simulink model "VHF_central_unit"  (R2024a)
settings: Solver=FixedStepDiscrete  StartTime=0.0  StopTime=10.0  FixedStep=0.001  RelTol=1e-3  EnableMultiTasking=on
PreLoadFcn:
  | try
  | MDL_install;
  | catch
  | end
InitFcn:
  | EcoCoder_PreCheckLic();
undefined symbols (not defined in the file or in its folder): C_ROTSPD_ZERO, C_SOC_ZERO, h, km, s, V
libraries: CoderSF_BSW_Libs x222, SF_CanService_Libs x16, CoderSF_ADC2Volt_Libs x6, CoderSF_6AxisMEMS_Libs x6, canmsglib x3, EV_ASWLibs x2, simulink x2, Chassis_stability_controllers x1, CoderSF_KeyCycle_Libs x1
(part 2 of 4)

== system VHF_central_unit/General Power Control1/Control KeyCycle ==
  flgKeyon_raw : Inport
  function : TriggerPort  TriggerType=function-call  VariantControl=(inherit)
  KeyCycle to Reset : CoderSF_KeyCycle_Libs/KeyCycle to Reset
  Read Calibration1 : CoderSF_BSW_Libs/Calibration & Measurement/Read Calibration  variable_name=PwrMCU_tResetDbncKeyOffFall_val  variable_value=0.2  variable_type=single  variable_min=[]  variable_max=[]  unitStr=s  descStr=""
      settings: AttributesFormatString=value:%<variable_value> type:%<variable_type> max:%<variable_max> Min:%<variable_min>
  Read Calibration2 : CoderSF_BSW_Libs/Calibration & Measurement/Read Calibration  variable_name=PwrMCU_tResetDbncKeyOffRise_val  variable_value=0.2  variable_type=single  variable_min=[]  variable_max=[]  unitStr=s  descStr=""
      settings: AttributesFormatString=value:%<variable_value> type:%<variable_type> max:%<variable_max> Min:%<variable_min>
  Read Calibration3 : CoderSF_BSW_Libs/Calibration & Measurement/Read Calibration  variable_name=PwrMCU_flgResetSWEn_val  variable_value=0  variable_type=boolean  variable_min=[]  variable_max=[]  unitStr=""  descStr=""
      settings: AttributesFormatString=value:%<variable_value> type:%<variable_type> max:%<variable_max> Min:%<variable_min>
  flgReset : Outport
  wires:
  flgKeyon_raw/1 -> KeyCycle to Reset/1
  Read Calibration2/1 -> KeyCycle to Reset/4
  Read Calibration3/1 -> KeyCycle to Reset/2
  Read Calibration1/1 -> KeyCycle to Reset/3
  KeyCycle to Reset/1 -> flgReset/1

== system VHF_central_unit/General Power Control1/Control Restore All NVM Data ==
  flgEnNVMRestore : Inport
  function : TriggerPort  TriggerType=function-call  VariantControl=(inherit)
  Restore All NVM Data Hold : CoderSF_BSW_Libs/Non-volatile Memory Blocks/Restore All NVM Data Hold
  wires:
  flgEnNVMRestore/1 -> Restore All NVM Data Hold/Enable

== system VHF_central_unit/General Power Control1/Debounce KeyOn ==
  flgKeyOnRaw : Inport
  function : TriggerPort  TriggerType=function-call  VariantControl=(inherit)
  Falling Edge Debounce1 : CoderSF_BSW_Libs/Application Base Blocks/Falling Edge Debounce  ic=off
  Read Calibration3 : CoderSF_BSW_Libs/Calibration & Measurement/Read Calibration  variable_name=PwrMCU_tDbncKeyOn_val  variable_value=0.05  variable_type=single  variable_min=[]  variable_max=[]  unitStr=s  descStr=""
      settings: AttributesFormatString=value:%<variable_value> type:%<variable_type> max:%<variable_max> Min:%<variable_min>
  Read Calibration5 : CoderSF_BSW_Libs/Calibration & Measurement/Read Calibration  variable_name=PwrMCU_tDbncKeyOff_val  variable_value=0.05  variable_type=single  variable_min=[]  variable_max=[]  unitStr=s  descStr=""
      settings: AttributesFormatString=value:%<variable_value> type:%<variable_type> max:%<variable_max> Min:%<variable_min>
  Rising Edge Debounce : CoderSF_BSW_Libs/Application Base Blocks/Rising Edge Debounce  ic=off
  Write and Read Measurement : CoderSF_BSW_Libs/Calibration & Measurement/Write and Read Measurement  variable_name=PwrMCU_flgKeyOnDbnc  variable_value=0  variable_type=boolean  numD=1  unitStr=""  descStr=""
      settings: AttributesFormatString=type:%<variable_type> Dimensions:%<numD>
  PwrMCU_flgKeyOnDbnc : Outport
  wires:
  Read Calibration5/1 -> Falling Edge Debounce1/1
  Read Calibration3/1 -> Rising Edge Debounce/1
  Rising Edge Debounce/1 -> Falling Edge Debounce1/2
  Falling Edge Debounce1/1 -> Write and Read Measurement/1
  Write and Read Measurement/1 -> PwrMCU_flgKeyOnDbnc/1  "PwrMCU_flgKeyOnDbnc"
  flgKeyOnRaw/1 -> Rising Edge Debounce/2

== system VHF_central_unit/General Power Control1/Enable Restore And Store NVM ==
  flgKeyon : Inport
  flgEnRestoreStoreNVM_val : Inport  Port=2
  function : TriggerPort  TriggerType=function-call  VariantControl=(inherit)
  Constant2 : Constant  Value=0
  Logical Operator2 : Logic  AllPortsSameDT=off  OutDataTypeStr=boolean
  SR Flip Flop : CoderSF_BSW_Libs/Application Base Blocks/SR Flip Flop
  Terminator : Terminator
  flgEnStoreNVM : Outport
  wires:
  flgKeyon/1 -> SR Flip Flop/1
  Logical Operator2/1 -> flgEnStoreNVM/1
  Constant2/1 -> SR Flip Flop/2
  SR Flip Flop/1 -> Logical Operator2/1
  flgEnRestoreStoreNVM_val/1 -> Logical Operator2/2
  SR Flip Flop/2 -> Terminator/1

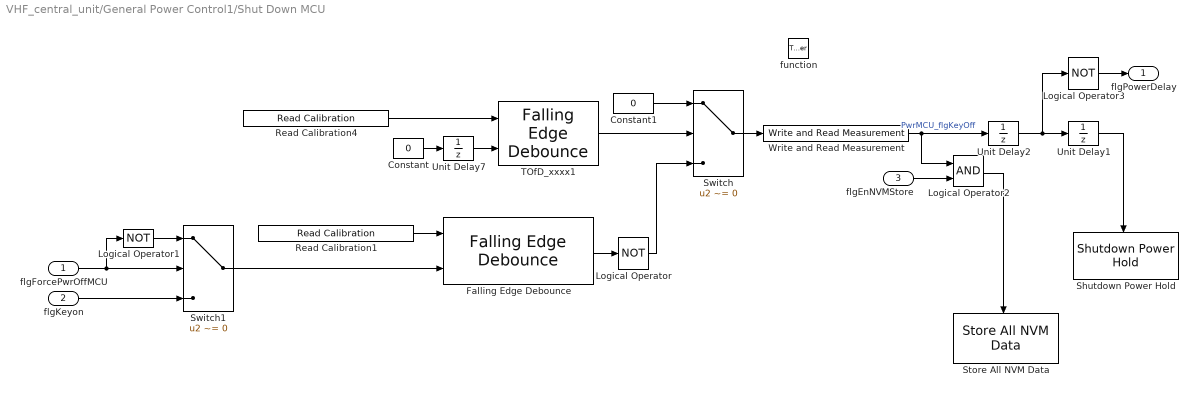
== system VHF_central_unit/General Power Control1/Shut Down MCU ==
  flgForcePwrOffMCU : Inport
  flgKeyon : Inport  Port=2
  flgEnNVMStore : Inport  Port=3
  function : TriggerPort  TriggerType=function-call  VariantControl=(inherit)
  Constant : Constant  Value=0
  Constant1 : Constant  Value=0  OutDataTypeStr=Inherit: Inherit via back propagation  SampleTime=-1
  Falling Edge Debounce : CoderSF_BSW_Libs/Application Base Blocks/Falling Edge Debounce  ic=off
  Logical Operator : Logic  Operator=NOT  AllPortsSameDT=off  OutDataTypeStr=boolean
  Logical Operator1 : Logic  Operator=NOT  AllPortsSameDT=off  OutDataTypeStr=boolean
  Logical Operator2 : Logic  AllPortsSameDT=off  OutDataTypeStr=boolean
  Logical Operator3 : Logic  Operator=NOT  AllPortsSameDT=off  OutDataTypeStr=boolean
  Read Calibration1 : CoderSF_BSW_Libs/Calibration & Measurement/Read Calibration  variable_name=PwrMCU_tShutDownDelay_val  variable_value=0.5  variable_type=single  variable_min=[]  variable_max=[]  unitStr=s  descStr=""
      settings: AttributesFormatString=value:%<variable_value> type:%<variable_type> max:%<variable_max> Min:%<variable_min>
  Read Calibration4 : CoderSF_BSW_Libs/Calibration & Measurement/Read Calibration  variable_name=PwrMCU_tWaitKeyOn_val  variable_value=0.2  variable_type=single  variable_min=[]  variable_max=[]  unitStr=s  descStr=""
      settings: AttributesFormatString=value:%<variable_value> type:%<variable_type> max:%<variable_max> Min:%<variable_min>
  Shutdown Power Hold : CoderSF_BSW_Libs/System Management Blocks/Shutdown Power Hold  tWait_ms=500
  Store All NVM Data : CoderSF_BSW_Libs/Non-volatile Memory Blocks/Store All NVM Data  TriggerTypeSet=rising
  Switch : Switch  Criteria=u2 ~= 0  SaturateOnIntegerOverflow=off  InputSameDT=off
  Switch1 : Switch  Criteria=u2 ~= 0  SaturateOnIntegerOverflow=off  InputSameDT=off
  TOfD_xxxx1 : CoderSF_BSW_Libs/Application Base Blocks/Falling Edge Debounce  ic=off
  Unit Delay1 : UnitDelay  SampleTime=-1
      settings: AttributesFormatString=InitialCondition:%<InitialCondition>
  Unit Delay2 : UnitDelay  SampleTime=-1
      settings: AttributesFormatString=InitialCondition:%<InitialCondition>
  Unit Delay7 : UnitDelay  InitialCondition=1  SampleTime=-1
      settings: AttributesFormatString=InitialCondition:%<InitialCondition>
  Write and Read Measurement : CoderSF_BSW_Libs/Calibration & Measurement/Write and Read Measurement  variable_name=PwrMCU_flgKeyOff  variable_value=0  variable_type=boolean  numD=1  unitStr=""  descStr=""
      settings: AttributesFormatString=type:%<variable_type> Dimensions:%<numD>
  flgPowerDelay : Outport
  wires:
  Logical Operator3/1 -> flgPowerDelay/1
  Unit Delay2/1 -> Unit Delay1/1, Logical Operator3/1
  Read Calibration1/1 -> Falling Edge Debounce/1
  Logical Operator/1 -> Switch/3
  Falling Edge Debounce/1 -> Logical Operator/1
  Constant1/1 -> Switch/1
  TOfD_xxxx1/1 -> Switch/2
  flgKeyon/1 -> Switch1/3
  Read Calibration4/1 -> TOfD_xxxx1/1
  Unit Delay7/1 -> TOfD_xxxx1/2
  Constant/1 -> Unit Delay7/1
  flgForcePwrOffMCU/1 -> Switch1/2, Logical Operator1/1
  Switch1/1 -> Falling Edge Debounce/2
  Logical Operator1/1 -> Switch1/1
  Unit Delay1/1 -> Shutdown Power Hold/Enable
  Switch/1 -> Write and Read Measurement/1
  Logical Operator2/1 -> Store All NVM Data/Trigger
  flgEnNVMStore/1 -> Logical Operator2/2
  Write and Read Measurement/1 -> Unit Delay2/1, Logical Operator2/1  "PwrMCU_flgKeyOff"

== system VHF_central_unit/Get wake-up signal1/Get wake-up signal ==
  function : TriggerPort  TriggerType=function-call  VariantControl=(inherit)
  ADC Value To Volt : CoderSF_ADC2Volt_Libs/ADC Value To Volt  ResValue=12  RefValue=5  TypeOut=Inherit: Inherit via back propagation  WithDiv=on  DivValue=3.48  SerValue=22
  Hysteresis : CoderSF_BSW_Libs/Application Base Blocks/Hysteresis
  Logical Operator : Logic  Operator=OR  Inputs=3  AllPortsSameDT=off  OutDataTypeStr=boolean
  Read ADC Value : CoderSF_BSW_Libs/ADC/Read ADC Value  channel=AI_KEYON
  Read Calibration1 : CoderSF_BSW_Libs/Calibration & Measurement/Read Calibration  variable_name=PwrMCU_voltKeyOnHysteresis_val  variable_value=3  variable_type=single  variable_min=[]  variable_max=[]  unitStr=s  descStr=""
      settings: AttributesFormatString=value:%<variable_value> type:%<variable_type> max:%<variable_max> Min:%<variable_min>
  Read Calibration5 : CoderSF_BSW_Libs/Calibration & Measurement/Read Calibration  variable_name=PwrMCU_voltKeyOffThreshold_val  variable_value=2  variable_type=single  variable_min=[]  variable_max=[]  unitStr=s  descStr=""
      settings: AttributesFormatString=value:%<variable_value> type:%<variable_type> max:%<variable_max> Min:%<variable_min>
  Switch Input1 : CoderSF_BSW_Libs/Digital I//O/Switch Input  portNum=DI_WAKE1
  Switch Input2 : CoderSF_BSW_Libs/Digital I//O/Switch Input  portNum=DI_WAKE2
  Write and Read Measurement : CoderSF_BSW_Libs/Calibration & Measurement/Write and Read Measurement  variable_name=PwrMCU_voltKeyOn  variable_value=0  variable_type=single  numD=1  unitStr=V  descStr=""
      settings: AttributesFormatString=type:%<variable_type> Dimensions:%<numD>
  Write and Read Measurement1 : CoderSF_BSW_Libs/Calibration & Measurement/Write and Read Measurement  variable_name=PwrMCU_adKeyOn  variable_value=0  variable_type=uint16  numD=1  unitStr=""  descStr=""
      settings: AttributesFormatString=type:%<variable_type> Dimensions:%<numD>
  Write and Read Measurement2 : CoderSF_BSW_Libs/Calibration & Measurement/Write and Read Measurement  variable_name=PwrMCU_flgKeyOnRead  variable_value=0  variable_type=boolean  numD=1  unitStr=""  descStr=""
      settings: AttributesFormatString=type:%<variable_type> Dimensions:%<numD>
  PwrVCU_flgKeyOn : Outport
  wires:
  Logical Operator/1 -> PwrVCU_flgKeyOn/1
  Hysteresis/1 -> Write and Read Measurement2/1
  Switch Input1/1 -> Logical Operator/2
  Switch Input2/1 -> Logical Operator/3
  Read ADC Value/1 -> Write and Read Measurement1/1
  ADC Value To Volt/1 -> Write and Read Measurement/1
  Read Calibration5/1 -> Hysteresis/3
  Read Calibration1/1 -> Hysteresis/1
  Write and Read Measurement/1 -> Hysteresis/2  "PwrMCU_voltKeyOn"
  Write and Read Measurement1/1 -> ADC Value To Volt/1  "PwrMCU_adKeyOn"
  Write and Read Measurement2/1 -> Logical Operator/1  "PwrMCU_flgKeyOnRead"

== system VHF_central_unit/MEMS sensor/Sensor Self Test ==
  function : TriggerPort  TriggerType=function-call  VariantControl=(inherit)
  6-Axis MEMS Sensor Self Test : CoderSF_6AxisMEMS_Libs/6-Axis MEMS Sensor/6-Axis MEMS Sensor Self Test
  "Write Fixed NVM " : CoderSF_BSW_Libs/Non-volatile Memory Blocks/Write Fixed NVM   data_name=Fnvm_Sensor_stSelfTest
  Write and Read Measurement : CoderSF_BSW_Libs/Calibration & Measurement/Write and Read Measurement  variable_name=Sensor_stSelfTest  variable_value=0  variable_type=uint8  numD=1  unitStr=""  descStr=""
      settings: AttributesFormatString=type:%<variable_type> Dimensions:%<numD>
  wires:
  6-Axis MEMS Sensor Self Test/1 -> Write and Read Measurement/1
  Write and Read Measurement/1 -> "Write Fixed NVM "/1  "Sensor_stSelfTest"

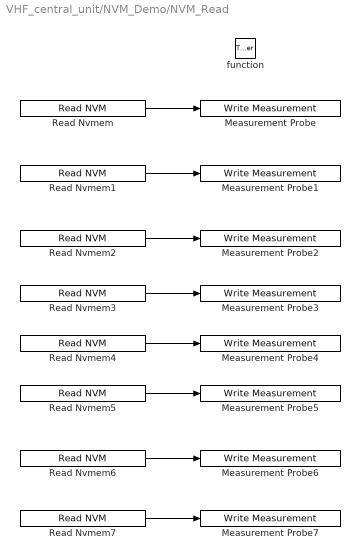
== system VHF_central_unit/NVM_Demo/NVM_Read ==
  function : TriggerPort  TriggerType=function-call  VariantControl=(inherit)
  Measurement Probe : CoderSF_BSW_Libs/Calibration & Measurement/Write Measurement  variable_name=ASW_V_single  variable_value=0  variable_type=single  numD=1  unitStr=""  descStr=""
      settings: AttributesFormatString=value:%<variable_value> type:%<variable_type>
  Measurement Probe1 : CoderSF_BSW_Libs/Calibration & Measurement/Write Measurement  variable_name=ASW_V_int8  variable_value=0  variable_type=int8  numD=1  unitStr=""  descStr=""
      settings: AttributesFormatString=value:%<variable_value> type:%<variable_type>
  Measurement Probe2 : CoderSF_BSW_Libs/Calibration & Measurement/Write Measurement  variable_name=ASW_V_uint8  variable_value=0  variable_type=uint8  numD=1  unitStr=""  descStr=""
      settings: AttributesFormatString=value:%<variable_value> type:%<variable_type>
  Measurement Probe3 : CoderSF_BSW_Libs/Calibration & Measurement/Write Measurement  variable_name=ASW_V_int16  variable_value=0  variable_type=int16  numD=1  unitStr=""  descStr=""
      settings: AttributesFormatString=value:%<variable_value> type:%<variable_type>
  Measurement Probe4 : CoderSF_BSW_Libs/Calibration & Measurement/Write Measurement  variable_name=ASW_V_uint16  variable_value=0  variable_type=uint16  numD=1  unitStr=""  descStr=""
      settings: AttributesFormatString=value:%<variable_value> type:%<variable_type>
  Measurement Probe5 : CoderSF_BSW_Libs/Calibration & Measurement/Write Measurement  variable_name=ASW_V_int32  variable_value=0  variable_type=int32  numD=1  unitStr=""  descStr=""
      settings: AttributesFormatString=value:%<variable_value> type:%<variable_type>
  Measurement Probe6 : CoderSF_BSW_Libs/Calibration & Measurement/Write Measurement  variable_name=ASW_V_uint32  variable_value=0  variable_type=uint32  numD=1  unitStr=""  descStr=""
      settings: AttributesFormatString=value:%<variable_value> type:%<variable_type>
  Measurement Probe7 : CoderSF_BSW_Libs/Calibration & Measurement/Write Measurement  variable_name=ASW_V_boolean  variable_value=0  variable_type=boolean  numD=1  unitStr=""  descStr=""
      settings: AttributesFormatString=value:%<variable_value> type:%<variable_type>
  Read Nvmem : CoderSF_BSW_Libs/Non-volatile Memory Blocks/Read NVM  variable_name=ASW_Nvm_single  variable_type=Inherit from 'Variable definition'
      settings: AttributesFormatString=type:%<variable_type>
  Read Nvmem1 : CoderSF_BSW_Libs/Non-volatile Memory Blocks/Read NVM  variable_name=ASW_Nvm_int8  variable_type=Inherit from 'Variable definition'
      settings: AttributesFormatString=type:%<variable_type>
  Read Nvmem2 : CoderSF_BSW_Libs/Non-volatile Memory Blocks/Read NVM  variable_name=ASW_Nvm_uint8  variable_type=Inherit from 'Variable definition'
      settings: AttributesFormatString=type:%<variable_type>
  Read Nvmem3 : CoderSF_BSW_Libs/Non-volatile Memory Blocks/Read NVM  variable_name=ASW_Nvm_int16  variable_type=Inherit from 'Variable definition'
      settings: AttributesFormatString=type:%<variable_type>
  Read Nvmem4 : CoderSF_BSW_Libs/Non-volatile Memory Blocks/Read NVM  variable_name=ASW_Nvm_uint16  variable_type=Inherit from 'Variable definition'
      settings: AttributesFormatString=type:%<variable_type>
  Read Nvmem5 : CoderSF_BSW_Libs/Non-volatile Memory Blocks/Read NVM  variable_name=ASW_Nvm_int32  variable_type=Inherit from 'Variable definition'
      settings: AttributesFormatString=type:%<variable_type>
  Read Nvmem6 : CoderSF_BSW_Libs/Non-volatile Memory Blocks/Read NVM  variable_name=ASW_Nvm_uint32  variable_type=Inherit from 'Variable definition'
      settings: AttributesFormatString=type:%<variable_type>
  Read Nvmem7 : CoderSF_BSW_Libs/Non-volatile Memory Blocks/Read NVM  variable_name=ASW_Nvm_boolean  variable_type=Inherit from 'Variable definition'
      settings: AttributesFormatString=type:%<variable_type>
  wires:
  Read Nvmem7/1 -> Measurement Probe7/1
  Read Nvmem6/1 -> Measurement Probe6/1
  Read Nvmem5/1 -> Measurement Probe5/1
  Read Nvmem4/1 -> Measurement Probe4/1
  Read Nvmem3/1 -> Measurement Probe3/1
  Read Nvmem2/1 -> Measurement Probe2/1
  Read Nvmem1/1 -> Measurement Probe1/1
  Read Nvmem/1 -> Measurement Probe/1

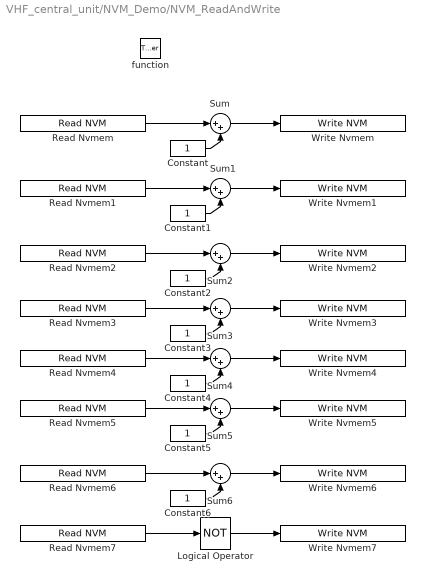
== system VHF_central_unit/NVM_Demo/NVM_ReadAndWrite ==
  function : TriggerPort  TriggerType=function-call  VariantControl=(inherit)
  Constant{,1..6} (7 alike) : Constant  OutDataTypeStr=Inherit: Inherit via back propagation  SampleTime=-1
  Logical Operator : Logic  Operator=NOT  AllPortsSameDT=off  OutDataTypeStr=boolean
  Read Nvmem : CoderSF_BSW_Libs/Non-volatile Memory Blocks/Read NVM  variable_name=ASW_Nvm_single  variable_type=Inherit from 'Variable definition'
      settings: AttributesFormatString=type:%<variable_type>
  Read Nvmem1 : CoderSF_BSW_Libs/Non-volatile Memory Blocks/Read NVM  variable_name=ASW_Nvm_int8  variable_type=Inherit from 'Variable definition'
      settings: AttributesFormatString=type:%<variable_type>
  Read Nvmem2 : CoderSF_BSW_Libs/Non-volatile Memory Blocks/Read NVM  variable_name=ASW_Nvm_uint8  variable_type=Inherit from 'Variable definition'
      settings: AttributesFormatString=type:%<variable_type>
  Read Nvmem3 : CoderSF_BSW_Libs/Non-volatile Memory Blocks/Read NVM  variable_name=ASW_Nvm_int16  variable_type=Inherit from 'Variable definition'
      settings: AttributesFormatString=type:%<variable_type>
  Read Nvmem4 : CoderSF_BSW_Libs/Non-volatile Memory Blocks/Read NVM  variable_name=ASW_Nvm_uint16  variable_type=Inherit from 'Variable definition'
      settings: AttributesFormatString=type:%<variable_type>
  Read Nvmem5 : CoderSF_BSW_Libs/Non-volatile Memory Blocks/Read NVM  variable_name=ASW_Nvm_int32  variable_type=Inherit from 'Variable definition'
      settings: AttributesFormatString=type:%<variable_type>
  Read Nvmem6 : CoderSF_BSW_Libs/Non-volatile Memory Blocks/Read NVM  variable_name=ASW_Nvm_uint32  variable_type=Inherit from 'Variable definition'
      settings: AttributesFormatString=type:%<variable_type>
  Read Nvmem7 : CoderSF_BSW_Libs/Non-volatile Memory Blocks/Read NVM  variable_name=ASW_Nvm_boolean  variable_type=Inherit from 'Variable definition'
      settings: AttributesFormatString=type:%<variable_type>
  Sum{,1..6} (7 alike) : Sum  Inputs=|++
  Write Nvmem : CoderSF_BSW_Libs/Non-volatile Memory Blocks/Write NVM  variable_name=ASW_Nvm_single  flgDef=on  variable_value=0  variable_type=single  variable_numD=1  unitStr=""  descStr=""  EcoCoderBlockID=N001_NVMVDEF
      settings: AttributesFormatString=value:%<variable_value> type:%<variable_type> D:%<variable_numD>
  Write Nvmem1 : CoderSF_BSW_Libs/Non-volatile Memory Blocks/Write NVM  variable_name=ASW_Nvm_int8  flgDef=on  variable_value=0  variable_type=int8  variable_numD=1  unitStr=""  descStr=""  EcoCoderBlockID=N001_NVMVDEF
      settings: AttributesFormatString=value:%<variable_value> type:%<variable_type> D:%<variable_numD>
  Write Nvmem2 : CoderSF_BSW_Libs/Non-volatile Memory Blocks/Write NVM  variable_name=ASW_Nvm_uint8  flgDef=on  variable_value=0  variable_type=uint8  variable_numD=1  unitStr=""  descStr=""  EcoCoderBlockID=N001_NVMVDEF
      settings: AttributesFormatString=value:%<variable_value> type:%<variable_type> D:%<variable_numD>
  Write Nvmem3 : CoderSF_BSW_Libs/Non-volatile Memory Blocks/Write NVM  variable_name=ASW_Nvm_int16  flgDef=on  variable_value=0  variable_type=int16  variable_numD=1  unitStr=""  descStr=""  EcoCoderBlockID=N001_NVMVDEF
      settings: AttributesFormatString=value:%<variable_value> type:%<variable_type> D:%<variable_numD>
  Write Nvmem4 : CoderSF_BSW_Libs/Non-volatile Memory Blocks/Write NVM  variable_name=ASW_Nvm_uint16  flgDef=on  variable_value=0  variable_type=uint16  variable_numD=1  unitStr=""  descStr=""  EcoCoderBlockID=N001_NVMVDEF
      settings: AttributesFormatString=value:%<variable_value> type:%<variable_type> D:%<variable_numD>
  Write Nvmem5 : CoderSF_BSW_Libs/Non-volatile Memory Blocks/Write NVM  variable_name=ASW_Nvm_int32  flgDef=on  variable_value=0  variable_type=int32  variable_numD=1  unitStr=""  descStr=""  EcoCoderBlockID=N001_NVMVDEF
      settings: AttributesFormatString=value:%<variable_value> type:%<variable_type> D:%<variable_numD>
  Write Nvmem6 : CoderSF_BSW_Libs/Non-volatile Memory Blocks/Write NVM  variable_name=ASW_Nvm_uint32  flgDef=on  variable_value=0  variable_type=uint32  variable_numD=1  unitStr=""  descStr=""  EcoCoderBlockID=N001_NVMVDEF
      settings: AttributesFormatString=value:%<variable_value> type:%<variable_type> D:%<variable_numD>
  Write Nvmem7 : CoderSF_BSW_Libs/Non-volatile Memory Blocks/Write NVM  variable_name=ASW_Nvm_boolean  flgDef=on  variable_value=0  variable_type=boolean  variable_numD=1  unitStr=""  descStr=""  EcoCoderBlockID=N001_NVMVDEF
      settings: AttributesFormatString=value:%<variable_value> type:%<variable_type> D:%<variable_numD>
  wires:
  Read Nvmem7/1 -> Logical Operator/1
  Logical Operator/1 -> Write Nvmem7/1
  Read Nvmem6/1 -> Sum6/1
  Constant6/1 -> Sum6/2
  Sum6/1 -> Write Nvmem6/1
  Read Nvmem5/1 -> Sum5/1
  Constant5/1 -> Sum5/2
  Sum5/1 -> Write Nvmem5/1
  Read Nvmem4/1 -> Sum4/1
  Constant4/1 -> Sum4/2
  Sum4/1 -> Write Nvmem4/1
  Read Nvmem3/1 -> Sum3/1
  Constant3/1 -> Sum3/2
  Sum3/1 -> Write Nvmem3/1
  Read Nvmem2/1 -> Sum2/1
  Constant2/1 -> Sum2/2
  Sum2/1 -> Write Nvmem2/1
  Read Nvmem1/1 -> Sum1/1
  Constant1/1 -> Sum1/2
  Sum1/1 -> Write Nvmem1/1
  Read Nvmem/1 -> Sum/1
  Constant/1 -> Sum/2
  Sum/1 -> Write Nvmem/1

== system VHF_central_unit/Set PowerDelay1/Set PowerDelay of Switch Internal  ==
  flgPowerDelay : Inport
  function : TriggerPort  TriggerType=function-call  VariantControl=(inherit)
  "Switch Internal " : CoderSF_BSW_Libs/Digital I//O/Switch Internal   portNum=PowerDelay
  wires:
  flgPowerDelay/1 -> "Switch Internal "/1

== system VHF_central_unit/Set Software Reset1/Set Software Reset ==
  flgReset : Inport
  function : TriggerPort  TriggerType=function-call  VariantControl=(inherit)
  Software Reset Hold : CoderSF_BSW_Libs/System Management Blocks/Software Reset Hold
  wires:
  flgReset/1 -> Software Reset Hold/Enable

== system VHF_central_unit/ASW_Demo/01  process input signals/01 process electrical supply input signals ==
  02 process electrical supply input signals : Subsystem  TreatAsAtomicUnit=on
      settings: RTWSystemCode=Nonreusable function
  Task_Call1 : CoderSF_BSW_Libs/Task Scheduler/Task Trigger  tasktimeIndex=Task_L20ms
  sigInEsmBatt_volt : Outport
  wires:
  02 process electrical supply input signals/1(sigInEsmBatt_volt) -> sigInEsmBatt_volt/1
  Task_Call1/1 -> 02 process electrical supply input signals/Trigger

== system VHF_central_unit/ASW_Demo/01  process input signals/02 process driver input signals ==
  01 link driver input signals : Subsystem
  02 process driver input signals : Subsystem
  Task_Call : CoderSF_BSW_Libs/Task Scheduler/Task Trigger  tasktimeIndex=Task_H10ms
  Task_Call2 : CoderSF_BSW_Libs/Task Scheduler/Task Trigger  tasktimeIndex=Task_L20ms
  Terminator : Terminator
  sigInDrvPedacc_pct : Outport
  wires:
  01 link driver input signals/1(sigInLinkDrvKey_flgOn) -> Terminator/1
  Task_Call/1 -> 01 link driver input signals/Trigger
  02 process driver input signals/1(sigInDrvPedacc_pct) -> sigInDrvPedacc_pct/1
  01 link driver input signals/3(sigInLinkDrvPedacc_volt2) -> 02 process driver input signals/2(sigInLinkDrvPedacc_volt2)
  01 link driver input signals/2(sigInLinkDrvPedacc_volt1) -> 02 process driver input signals/1(sigInLinkDrvPedacc_volt1)
  Task_Call2/1 -> 02 process driver input signals/Trigger

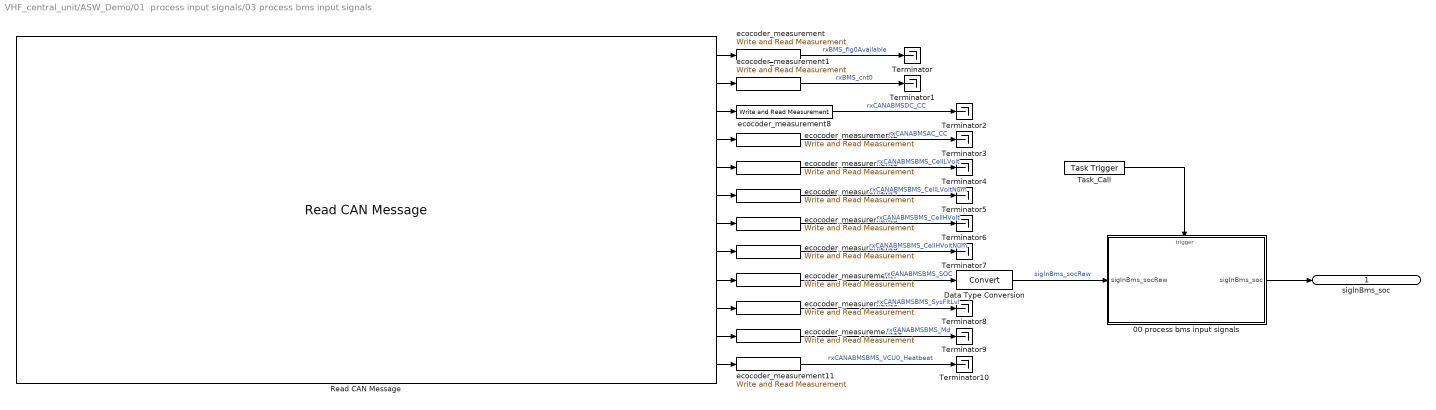
== system VHF_central_unit/ASW_Demo/01  process input signals/03 process bms input signals ==
  00 process bms input signals : Subsystem  TreatAsAtomicUnit=on
      settings: RTWSystemCode=Nonreusable function
  Data Type Conversion : DataTypeConversion  SaturateOnIntegerOverflow=off  RndMeth=Floor
  "Read CAN Message " : SF_CanService_Libs/Read CAN Message  typeCAN=Connected  channel=CAN_A  mEn=off  msgInfo=EcoCanM_Demo  msgItermStore=BMS_HCU_0  msgIterm=BMS_HCU_0  valid=on  stale=on  motoBit=off  setSignalName=off  flgCustomMonitorVariableRules=on  defineSignalName=off  prefixSignal='rxCANABMS'  flgValTest=off  flgNoFixed=on  flgInheritForNoFixed=on  tSample=Task_L10ms  modeCode=Parameterless
  Task_Call : CoderSF_BSW_Libs/Task Scheduler/Task Trigger  tasktimeIndex=Task_L20ms
  Terminator{,1..10} (11 alike) : Terminator
  ecocoder_measurement : CoderSF_BSW_Libs/Calibration & Measurement/Write and Read Measurement  variable_name=rxBMS_flg0Available  variable_value=0  variable_type=boolean  numD=1  unitStr=""  descStr=""
      settings: AttributesFormatString=value:%<variable_value> type:%<variable_type>
  ecocoder_measurement1 : CoderSF_BSW_Libs/Calibration & Measurement/Write and Read Measurement  variable_name=rxBMS_cnt0  variable_value=0  variable_type=uint32  numD=1  unitStr=""  descStr=""
      settings: AttributesFormatString=value:%<variable_value> type:%<variable_type>
  ecocoder_measurement10 : CoderSF_BSW_Libs/Calibration & Measurement/Write and Read Measurement  variable_name=rxCANABMSBMS_Md  variable_value=0  variable_type=uint8  numD=1  unitStr=""  descStr=""
      settings: AttributesFormatString=value:%<variable_value> type:%<variable_type>
  ecocoder_measurement11 : CoderSF_BSW_Libs/Calibration & Measurement/Write and Read Measurement  variable_name=rxCANABMSBMS_VCU0_Heatbeat  variable_value=0  variable_type=uint8  numD=1  unitStr=""  descStr=""
      settings: AttributesFormatString=value:%<variable_value> type:%<variable_type>
  ecocoder_measurement2 : CoderSF_BSW_Libs/Calibration & Measurement/Write and Read Measurement  variable_name=rxCANABMSAC_CC  variable_value=0  variable_type=boolean  numD=1  unitStr=""  descStr=""
      settings: AttributesFormatString=value:%<variable_value> type:%<variable_type>
  ecocoder_measurement3 : CoderSF_BSW_Libs/Calibration & Measurement/Write and Read Measurement  variable_name=rxCANABMSBMS_CellLVolt  variable_value=0  variable_type=single  numD=1  unitStr=""  descStr=""
      settings: AttributesFormatString=value:%<variable_value> type:%<variable_type>
  ecocoder_measurement4 : CoderSF_BSW_Libs/Calibration & Measurement/Write and Read Measurement  variable_name=rxCANABMSBMS_CellLVoltNum  variable_value=0  variable_type=uint8  numD=1  unitStr=""  descStr=""
      settings: AttributesFormatString=value:%<variable_value> type:%<variable_type>
  ecocoder_measurement5 : CoderSF_BSW_Libs/Calibration & Measurement/Write and Read Measurement  variable_name=rxCANABMSBMS_CellHVolt  variable_value=0  variable_type=single  numD=1  unitStr=""  descStr=""
      settings: AttributesFormatString=value:%<variable_value> type:%<variable_type>
  ecocoder_measurement6 : CoderSF_BSW_Libs/Calibration & Measurement/Write and Read Measurement  variable_name=rxCANABMSBMS_CellHVoltNum  variable_value=0  variable_type=uint8  numD=1  unitStr=""  descStr=""
      settings: AttributesFormatString=value:%<variable_value> type:%<variable_type>
  ecocoder_measurement7 : CoderSF_BSW_Libs/Calibration & Measurement/Write and Read Measurement  variable_name=rxCANABMSBMS_SOC  variable_value=0  variable_type=single  numD=1  unitStr=""  descStr=""
      settings: AttributesFormatString=value:%<variable_value> type:%<variable_type>
  ecocoder_measurement8 : CoderSF_BSW_Libs/Calibration & Measurement/Write and Read Measurement  variable_name=rxCANABMSDC_CC  variable_value=0  variable_type=boolean  numD=1  unitStr=""  descStr=""
      settings: AttributesFormatString=value:%<variable_value> type:%<variable_type>
  ecocoder_measurement9 : CoderSF_BSW_Libs/Calibration & Measurement/Write and Read Measurement  variable_name=rxCANABMSBMS_SysFltLvl  variable_value=0  variable_type=uint8  numD=1  unitStr=""  descStr=""
      settings: AttributesFormatString=value:%<variable_value> type:%<variable_type>
  sigInBms_soc : Outport
  wires:
  ecocoder_measurement11/1 -> Terminator10/1  "rxCANABMSBMS_VCU0_Heatbeat"
  ecocoder_measurement10/1 -> Terminator9/1  "rxCANABMSBMS_Md"
  ecocoder_measurement9/1 -> Terminator8/1  "rxCANABMSBMS_SysFltLvl"
  ecocoder_measurement7/1 -> Data Type Conversion/1  "rxCANABMSBMS_SOC"
  ecocoder_measurement6/1 -> Terminator7/1  "rxCANABMSBMS_CellHVoltNum"
  ecocoder_measurement5/1 -> Terminator6/1  "rxCANABMSBMS_CellHVolt"
  ecocoder_measurement4/1 -> Terminator5/1  "rxCANABMSBMS_CellLVoltNum"
  ecocoder_measurement3/1 -> Terminator4/1  "rxCANABMSBMS_CellLVolt"
  ecocoder_measurement2/1 -> Terminator3/1  "rxCANABMSAC_CC"
  ecocoder_measurement8/1 -> Terminator2/1  "rxCANABMSDC_CC"
  ecocoder_measurement1/1 -> Terminator1/1  "rxBMS_cnt0"
  ecocoder_measurement/1 -> Terminator/1  "rxBMS_flg0Available"
  "Read CAN Message "/10 -> ecocoder_measurement9/1
  "Read CAN Message "/12 -> ecocoder_measurement11/1
  "Read CAN Message "/11 -> ecocoder_measurement10/1
  "Read CAN Message "/5 -> ecocoder_measurement3/1
  "Read CAN Message "/3 -> ecocoder_measurement8/1
  "Read CAN Message "/2 -> ecocoder_measurement1/1
  "Read CAN Message "/4 -> ecocoder_measurement2/1
  "Read CAN Message "/1 -> ecocoder_measurement/1
  "Read CAN Message "/8 -> ecocoder_measurement6/1
  "Read CAN Message "/7 -> ecocoder_measurement5/1
  "Read CAN Message "/6 -> ecocoder_measurement4/1
  Data Type Conversion/1 -> 00 process bms input signals/1(sigInBms_socRaw)  "sigInBms_socRaw"
  "Read CAN Message "/9 -> ecocoder_measurement7/1
  00 process bms input signals/1(sigInBms_soc) -> sigInBms_soc/1
  Task_Call/1 -> 00 process bms input signals/Trigger

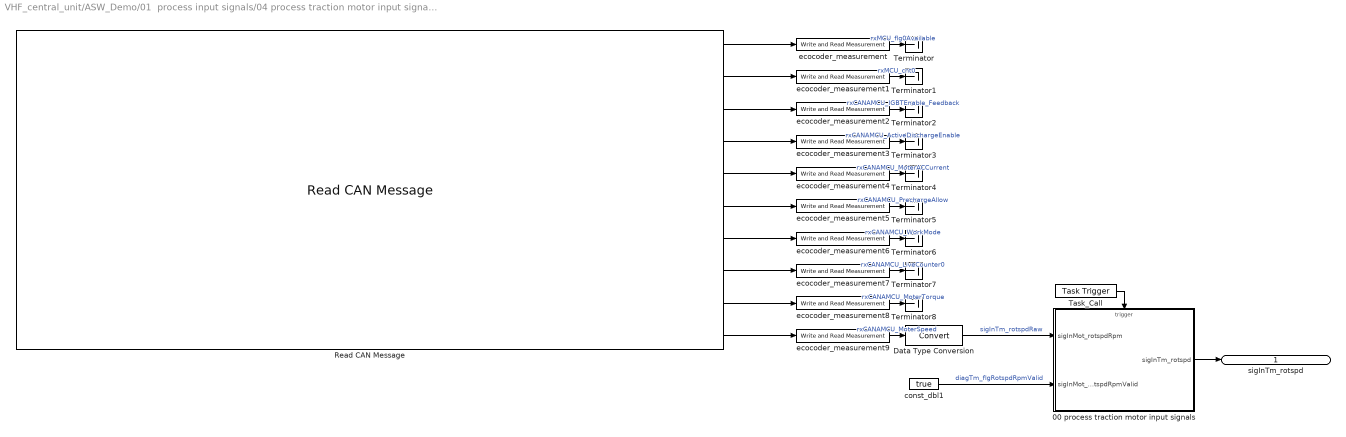
== system VHF_central_unit/ASW_Demo/01  process input signals/04 process traction motor input signals ==
  00 process traction motor input signals : Subsystem  TreatAsAtomicUnit=on
      settings: RTWSystemCode=Nonreusable function
  Data Type Conversion : DataTypeConversion  SaturateOnIntegerOverflow=off  RndMeth=Floor
  "Read CAN Message " : SF_CanService_Libs/Read CAN Message  typeCAN=Connected  channel=CAN_A  mEn=off  msgInfo=EcoCanM_Demo  msgItermStore=MCU_STATUS_1  msgIterm=MCU_STATUS_1  valid=on  stale=on  motoBit=off  setSignalName=off  flgCustomMonitorVariableRules=on  defineSignalName=off  prefixSignal='rxCANAMCU_'  flgValTest=off  flgNoFixed=on  flgInheritForNoFixed=on  tSample=Task_L20ms  modeCode=Parameterless
  Task_Call : CoderSF_BSW_Libs/Task Scheduler/Task Trigger  tasktimeIndex=Task_L20ms
  Terminator{,1..8} (9 alike) : Terminator
  const_dbl1 : Constant  Value=true  SampleTime=-1
  ecocoder_measurement : CoderSF_BSW_Libs/Calibration & Measurement/Write and Read Measurement  variable_name=rxMCU_flg0Available  variable_value=0  variable_type=boolean  numD=1  unitStr=""  descStr=""
      settings: AttributesFormatString=value:%<variable_value> type:%<variable_type>
  ecocoder_measurement1 : CoderSF_BSW_Libs/Calibration & Measurement/Write and Read Measurement  variable_name=rxMCU_cnt0  variable_value=0  variable_type=uint32  numD=1  unitStr=""  descStr=""
      settings: AttributesFormatString=value:%<variable_value> type:%<variable_type>
  ecocoder_measurement2 : CoderSF_BSW_Libs/Calibration & Measurement/Write and Read Measurement  variable_name=rxCANAMCU_IGBTEnable_Feedback  variable_value=0  variable_type=boolean  numD=1  unitStr=""  descStr=""
      settings: AttributesFormatString=value:%<variable_value> type:%<variable_type>
  ecocoder_measurement3 : CoderSF_BSW_Libs/Calibration & Measurement/Write and Read Measurement  variable_name=rxCANAMCU_ActiveDischargeEnable  variable_value=0  variable_type=boolean  numD=1  unitStr=""  descStr=""
      settings: AttributesFormatString=value:%<variable_value> type:%<variable_type>
  ecocoder_measurement4 : CoderSF_BSW_Libs/Calibration & Measurement/Write and Read Measurement  variable_name=rxCANAMCU_MoterACCurrent  variable_value=0  variable_type=single  numD=1  unitStr=""  descStr=""
      settings: AttributesFormatString=value:%<variable_value> type:%<variable_type>
  ecocoder_measurement5 : CoderSF_BSW_Libs/Calibration & Measurement/Write and Read Measurement  variable_name=rxCANAMCU_PrechargeAllow  variable_value=0  variable_type=boolean  numD=1  unitStr=""  descStr=""
      settings: AttributesFormatString=value:%<variable_value> type:%<variable_type>
  ecocoder_measurement6 : CoderSF_BSW_Libs/Calibration & Measurement/Write and Read Measurement  variable_name=rxCANAMCU_WorkMode  variable_value=0  variable_type=uint8  numD=1  unitStr=""  descStr=""
      settings: AttributesFormatString=value:%<variable_value> type:%<variable_type>
  ecocoder_measurement7 : CoderSF_BSW_Libs/Calibration & Measurement/Write and Read Measurement  variable_name=rxCANAMCU_LiveCounter0  variable_value=0  variable_type=uint8  numD=1  unitStr=""  descStr=""
      settings: AttributesFormatString=value:%<variable_value> type:%<variable_type>
  ecocoder_measurement8 : CoderSF_BSW_Libs/Calibration & Measurement/Write and Read Measurement  variable_name=rxCANAMCU_MoterTorque  variable_value=0  variable_type=single  numD=1  unitStr=""  descStr=""
      settings: AttributesFormatString=value:%<variable_value> type:%<variable_type>
  ecocoder_measurement9 : CoderSF_BSW_Libs/Calibration & Measurement/Write and Read Measurement  variable_name=rxCANAMCU_MoterSpeed  variable_value=0  variable_type=single  numD=1  unitStr=""  descStr=""
      settings: AttributesFormatString=value:%<variable_value> type:%<variable_type>
  sigInTm_rotspd : Outport
  wires:
  ecocoder_measurement8/1 -> Terminator8/1  "rxCANAMCU_MoterTorque"
  ecocoder_measurement7/1 -> Terminator7/1  "rxCANAMCU_LiveCounter0"
  ecocoder_measurement6/1 -> Terminator6/1  "rxCANAMCU_WorkMode"
  ecocoder_measurement5/1 -> Terminator5/1  "rxCANAMCU_PrechargeAllow"
  ecocoder_measurement4/1 -> Terminator4/1  "rxCANAMCU_MoterACCurrent"
  ecocoder_measurement3/1 -> Terminator3/1  "rxCANAMCU_ActiveDischargeEnable"
  ecocoder_measurement2/1 -> Terminator2/1  "rxCANAMCU_IGBTEnable_Feedback"
  "Read CAN Message "/4 -> ecocoder_measurement3/1
  "Read CAN Message "/5 -> ecocoder_measurement4/1
  "Read CAN Message "/3 -> ecocoder_measurement2/1
  "Read CAN Message "/7 -> ecocoder_measurement6/1
  "Read CAN Message "/6 -> ecocoder_measurement5/1
  "Read CAN Message "/8 -> ecocoder_measurement7/1
  "Read CAN Message "/9 -> ecocoder_measurement8/1
  "Read CAN Message "/10 -> ecocoder_measurement9/1
  "Read CAN Message "/1 -> ecocoder_measurement/1
  "Read CAN Message "/2 -> ecocoder_measurement1/1
  ecocoder_measurement1/1 -> Terminator1/1  "rxMCU_cnt0"
  ecocoder_measurement/1 -> Terminator/1  "rxMCU_flg0Available"
  Data Type Conversion/1 -> 00 process traction motor input signals/1(sigInMot_rotspdRpm)  "sigInTm_rotspdRaw"
  const_dbl1/1 -> 00 process traction motor input signals/2(sigInMot_flgRotspdRpmValid)  "diagTm_flgRotspdRpmValid"
  00 process traction motor input signals/1(sigInTm_rotspd) -> sigInTm_rotspd/1
  Task_Call/1 -> 00 process traction motor input signals/Trigger
  ecocoder_measurement9/1 -> Data Type Conversion/1  "rxCANAMCU_MoterSpeed"

== system VHF_central_unit/ASW_Demo/02 vehicle motion request/01 driver torque demand ==
  sigInDrvPedacc_pct1 : Inport
  f : TriggerPort  TriggerType=function-call  VariantControl=(inherit)
  Switch : Switch  Criteria=u2 ~= 0  SaturateOnIntegerOverflow=off  InputSameDT=off
  ecocoder_calibration : CoderSF_BSW_Libs/Calibration & Measurement/Read Calibration  variable_name=vehDrv_flgCal_val  variable_value=0  variable_type=boolean  variable_min=[]  variable_max=[]  unitStr=""  descStr=""
      settings: AttributesFormatString=value:%<variable_value> type:%<variable_type> max:%<variable_max> Min:%<variable_min>
  ecocoder_calibration1 : CoderSF_BSW_Libs/Calibration & Measurement/Read Calibration  variable_name=vehDrv_linspd_val  variable_value=0  variable_type=single  variable_min=[]  variable_max=[]  unitStr=km/h  descStr=""
      settings: AttributesFormatString=value:%<variable_value> type:%<variable_type> max:%<variable_max> Min:%<variable_min>
  ecocoder_calibration2 : CoderSF_BSW_Libs/Calibration & Measurement/Read Calibration  variable_name=vehDrv_pct_val  variable_value=0  variable_type=single  variable_min=[]  variable_max=[]  unitStr=""  descStr=""
      settings: AttributesFormatString=value:%<variable_value> type:%<variable_type> max:%<variable_max> Min:%<variable_min>
  ecocoder_measurement : CoderSF_BSW_Libs/Calibration & Measurement/Write and Read Measurement  variable_name=vehDrv_linspd  variable_value=0  variable_type=single  numD=1  unitStr=km/h  descStr=""
      settings: AttributesFormatString=value:%<variable_value> type:%<variable_type>
  ecocoder_measurement1 : CoderSF_BSW_Libs/Calibration & Measurement/Write and Read Measurement  variable_name=vehDrv_pct  variable_value=0  variable_type=single  numD=1  unitStr=""  descStr=""
      settings: AttributesFormatString=value:%<variable_value> type:%<variable_type>
  ecocoder_measurement2 : CoderSF_BSW_Libs/Calibration & Measurement/Write and Read Measurement  variable_name=vehDrv_trqReq  variable_value=0  variable_type=single  numD=1  unitStr=Nm  descStr=""
      settings: AttributesFormatString=value:%<variable_value> type:%<variable_type>
  vehDrv_trqEcoTracMax_map : CoderSF_BSW_Libs/Calibration & Measurement/2-D Lookup Table  nam=vehDrv_trqEcoTracMax  breakpoint1_type=single  breakpoint1_data=[0 0.1 0.2 0.3 0.4 0.5 0.6 0.7 0.8 0.9 0.95 1]  breakpoint2_type=single  breakpoint2_data="[0 2 3 10  20 30 40 50 60 70 80 90 95 100 115 120]"  table_type=single  table_data=|
      | [0 0 0 0 0 0 0 0 0 0 0 0 0 0 0 0 ;
      | 0 200 441 439 437 435 433 431 429 427 425 423 421 419 417 415 ;
      | 0 202 461 459 457 455 453 451 449 447 445 443 441 439 437 435 ;
      | 0 204 565 560 555 550 545 540 535 530 525 520 515 510 505 500 ;
      | 0 206 614 611 608 605 602 599 596 593 590 587 584 581 578 575 ;
      | 0 208 678 677 676 675 674 673 672 671 670 669 668 667 666 665 ;
      | 0 210 784 781 778 775 772 769 766 763 760 757 754 751 748 745 ;
      | 0 212 956 954 952 950 948 946 944 942 940 938 936 934 932 930 ;
      | 0 214 1078 1077 1076 1075 1074 1073 1072 1071 1070 1069 1068 1067 1066 1065 ;
      | 0 216 1376 1374 1372 1370 1368 1366 1364 1362 1360 1358 1356 1354 1352 1350 ;
      | 0 218 1576 1574 1572 1570 1568 1566 1564 1562 1560 1558 1556 1554 1552 1550 ;
      | 0 220 1900 1900 1900 1900 1900 1900 1900 1900 1900 1900 1900 1900 1900 1900 ]
  vehDrv_trqReq1 : Outport
  wires:
  vehDrv_trqEcoTracMax_map/1 -> ecocoder_measurement2/1
  ecocoder_calibration1/1 -> ecocoder_measurement/1
  sigInDrvPedacc_pct1/1 -> Switch/3
  Switch/1 -> ecocoder_measurement1/1
  ecocoder_calibration/1 -> Switch/2
  ecocoder_calibration2/1 -> Switch/1
  ecocoder_measurement/1 -> vehDrv_trqEcoTracMax_map/2  "vehDrv_linspd"
  ecocoder_measurement1/1 -> vehDrv_trqEcoTracMax_map/1  "vehDrv_pct"
  ecocoder_measurement2/1 -> vehDrv_trqReq1/1  "vehDrv_trqReq"

== system VHF_central_unit/ASW_Demo/03 electrical supply management/02  electrical supply control ==
  sigInEsmBatt_volt : Inport
  Task_Call4 : CoderSF_BSW_Libs/Task Scheduler/Task Trigger  tasktimeIndex=Task_L20ms
  esmc : Subsystem  TreatAsAtomicUnit=on
  esmcDcdc_flgEn : Outport
  wires:
  Task_Call4/1 -> esmc/Trigger
  esmc/1(esmcDcdc_flgEn) -> esmcDcdc_flgEn/1
  sigInEsmBatt_volt/1 -> esmc/1(sigInEsmBatt_volt)

== system VHF_central_unit/ASW_Demo/04 powertrain control /02  Bms control ==
  sigInBms_soc : Inport
  02  Bms control : Subsystem
  pwrtrnBmscPack_flgConnReq : Outport
  wires:
  sigInBms_soc/1 -> 02  Bms control/1(pwrtrn_stVeh)
  02  Bms control/1(pwrtrnBmscPack_flgConnReq) -> pwrtrnBmscPack_flgConnReq/1

== system VHF_central_unit/ASW_Demo/04 powertrain control /03  traction motor control ==
  sigInTm_rotspd : Inport  Interpolate=off
  vehDrv_trqReq : Inport  Port=2
  Task_Call1 : CoderSF_BSW_Libs/Task Scheduler/Task Trigger  tasktimeIndex=Task_L20ms
  tmc : Subsystem
  pwrtrnTmc_trqCmd : Outport
  wires:
  Task_Call1/1 -> tmc/Trigger
  tmc/1(pwrtrnTmc_trqCmd) -> pwrtrnTmc_trqCmd/1
  sigInTm_rotspd/1 -> tmc/1(sigInTm_rotspd)
  vehDrv_trqReq/1 -> tmc/2(vehDrv_trqReq)

== system VHF_central_unit/ASW_Demo/05 thermal management/thrml ==
  f : TriggerPort  TriggerType=function-call  VariantControl=(inherit)
  Const : Constant  Value=false  SampleTime=-1
  thrmlFan_flgCoolLoSpdEn : Outport
  wires:
  Const/1 -> thrmlFan_flgCoolLoSpdEn/1  "thrmlFan_flgCoolLoSpdEn"

== system VHF_central_unit/ASW_Demo/06 process output signals/01 process electrical supply output signals ==
  esmcDcdc_flgEn : Inport
  01 process electrical supply output signals : Subsystem
  Task_Call4 : CoderSF_BSW_Libs/Task Scheduler/Task Trigger  tasktimeIndex=Task_L20ms
  wires:
  Task_Call4/1 -> 01 process electrical supply output signals/Trigger
  esmcDcdc_flgEn/1 -> 01 process electrical supply output signals/1(esmcDcdc_flgEn)

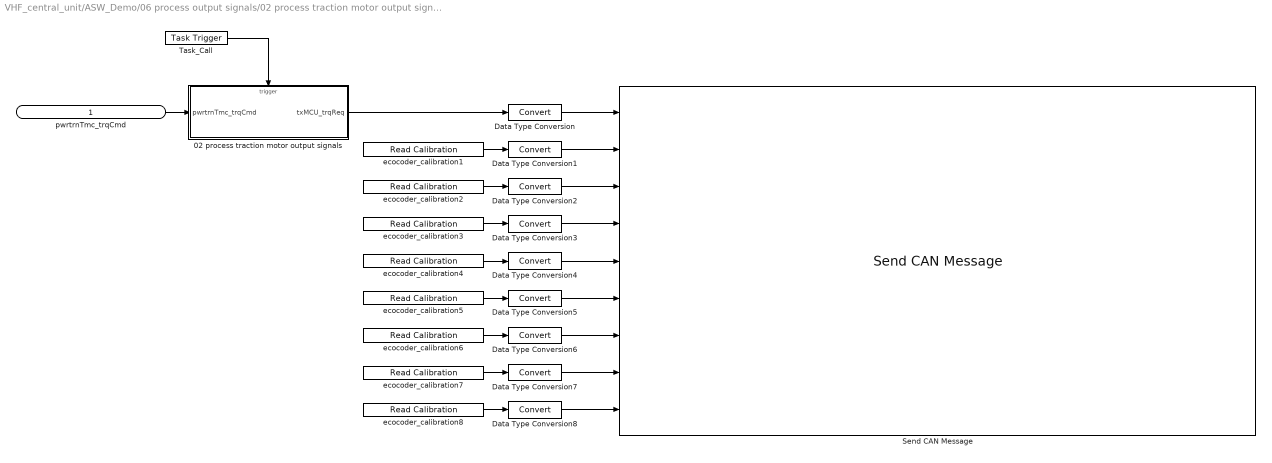
== system VHF_central_unit/ASW_Demo/06 process output signals/02 process traction motor output signals ==
  pwrtrnTmc_trqCmd : Inport  Interpolate=off
  02 process traction motor output signals : Subsystem
  Data Type Conversion{,1..8} (9 alike) : DataTypeConversion  SaturateOnIntegerOverflow=off  RndMeth=Floor
  Send CAN Message : SF_CanService_Libs/Send CAN Message   typeCAN=Connected  channel=CAN_A  mEn=off  msgInfo=EcoCanM_Demo  msgItermStore=HCU_COMMAND  msgIterm=HCU_COMMAND  motoBit=off  flgNoFixed=on  flgInheritForNoFixed=on  tSample=Task_L50ms  modeCode=Parameterless  modeRound=Zero
  Task_Call : CoderSF_BSW_Libs/Task Scheduler/Task Trigger  tasktimeIndex=Task_L20ms
  ecocoder_calibration1 : CoderSF_BSW_Libs/Calibration & Measurement/Read Calibration  variable_name=txHCUDemand_Torque_val  variable_value=-1  variable_type=single  variable_min=[]  variable_max=[]  unitStr=""  descStr=""
      settings: AttributesFormatString=value:%<variable_value> type:%<variable_type> max:%<variable_max> Min:%<variable_min>
  ecocoder_calibration2 : CoderSF_BSW_Libs/Calibration & Measurement/Read Calibration  variable_name=txHCUFaultReset_val  variable_value=1  variable_type=boolean  variable_min=[]  variable_max=[]  unitStr=""  descStr=""
      settings: AttributesFormatString=value:%<variable_value> type:%<variable_type> max:%<variable_max> Min:%<variable_min>
  ecocoder_calibration3 : CoderSF_BSW_Libs/Calibration & Measurement/Read Calibration  variable_name=txHCUDemand_LimitValid_val  variable_value=1  variable_type=single  variable_min=[]  variable_max=[]  unitStr=""  descStr=""
      settings: AttributesFormatString=value:%<variable_value> type:%<variable_type> max:%<variable_max> Min:%<variable_min>
  ecocoder_calibration4 : CoderSF_BSW_Libs/Calibration & Measurement/Read Calibration  variable_name=txHCUDemand_LimitLow_val  variable_value=0  variable_type=single  variable_min=[]  variable_max=[]  unitStr=""  descStr=""
      settings: AttributesFormatString=value:%<variable_value> type:%<variable_type> max:%<variable_max> Min:%<variable_min>
  ecocoder_calibration5 : CoderSF_BSW_Libs/Calibration & Measurement/Read Calibration  variable_name=txHCUDemand_LimitHigh_val  variable_value=0  variable_type=single  variable_min=[]  variable_max=[]  unitStr=""  descStr=""
      settings: AttributesFormatString=value:%<variable_value> type:%<variable_type> max:%<variable_max> Min:%<variable_min>
  ecocoder_calibration6 : CoderSF_BSW_Libs/Calibration & Measurement/Read Calibration  variable_name=txHCULive_Counter_val  variable_value=0  variable_type=uint8  variable_min=[]  variable_max=[]  unitStr=""  descStr=""
      settings: AttributesFormatString=value:%<variable_value> type:%<variable_type> max:%<variable_max> Min:%<variable_min>
  ecocoder_calibration7 : CoderSF_BSW_Libs/Calibration & Measurement/Read Calibration  variable_name=txHCUControl_Mode_val  variable_value=0  variable_type=uint8  variable_min=[]  variable_max=[]  unitStr=""  descStr=""
      settings: AttributesFormatString=value:%<variable_value> type:%<variable_type> max:%<variable_max> Min:%<variable_min>
  ecocoder_calibration8 : CoderSF_BSW_Libs/Calibration & Measurement/Read Calibration  variable_name=txHCUMCU_Enable_val  variable_value=1  variable_type=boolean  variable_min=[]  variable_max=[]  unitStr=""  descStr=""
      settings: AttributesFormatString=value:%<variable_value> type:%<variable_type> max:%<variable_max> Min:%<variable_min>
  wires:
  Data Type Conversion/1 -> Send CAN Message/1
  Data Type Conversion1/1 -> Send CAN Message/2
  Data Type Conversion3/1 -> Send CAN Message/4
  Data Type Conversion2/1 -> Send CAN Message/3
  Data Type Conversion8/1 -> Send CAN Message/9
  Data Type Conversion7/1 -> Send CAN Message/8
  Data Type Conversion6/1 -> Send CAN Message/7
  Data Type Conversion5/1 -> Send CAN Message/6
  Data Type Conversion4/1 -> Send CAN Message/5
  02 process traction motor output signals/1(txMCU_trqReq) -> Data Type Conversion/1
  ecocoder_calibration1/1 -> Data Type Conversion1/1
  ecocoder_calibration2/1 -> Data Type Conversion2/1
  ecocoder_calibration3/1 -> Data Type Conversion3/1
  ecocoder_calibration4/1 -> Data Type Conversion4/1
  ecocoder_calibration5/1 -> Data Type Conversion5/1
  ecocoder_calibration6/1 -> Data Type Conversion6/1
  ecocoder_calibration7/1 -> Data Type Conversion7/1
  ecocoder_calibration8/1 -> Data Type Conversion8/1
  Task_Call/1 -> 02 process traction motor output signals/Trigger
  pwrtrnTmc_trqCmd/1 -> 02 process traction motor output signals/1(pwrtrnTmc_trqCmd)

== system VHF_central_unit/ASW_Demo/06 process output signals/03 process bms output signals ==
  pwrtrnBmscPack_flgConnReq : Inport
  03 process bms output signals : Subsystem
  Data Type Conversion10 : DataTypeConversion  SaturateOnIntegerOverflow=off  RndMeth=Floor
  Data Type Conversion11 : DataTypeConversion  SaturateOnIntegerOverflow=off  RndMeth=Floor
  Data Type Conversion9 : DataTypeConversion  SaturateOnIntegerOverflow=off  RndMeth=Floor
  "Send CAN Message " : SF_CanService_Libs/Send CAN Message   typeCAN=Connected  channel=CAN_A  mEn=off  msgInfo=EcoCanM_Demo  msgItermStore=HCU_BMS_0  msgIterm=HCU_BMS_0  motoBit=off  flgNoFixed=on  flgInheritForNoFixed=on  tSample=Task_L10ms  modeCode=Parameterless  modeRound=Zero
  Task_Call : CoderSF_BSW_Libs/Task Scheduler/Task Trigger  tasktimeIndex=Task_L20ms
  ecocoder_calibration11 : CoderSF_BSW_Libs/Calibration & Measurement/Read Calibration  variable_name=txVCU_BMS0_Heartbeat_val  variable_value=1  variable_type=uint8  variable_min=[]  variable_max=[]  unitStr=""  descStr=""
      settings: AttributesFormatString=value:%<variable_value> type:%<variable_type> max:%<variable_max> Min:%<variable_min>
  ecocoder_calibration9 : CoderSF_BSW_Libs/Calibration & Measurement/Read Calibration  variable_name=txVCU_ChrageRlyStatus_val  variable_value=1  variable_type=boolean  variable_min=[]  variable_max=[]  unitStr=""  descStr=""
      settings: AttributesFormatString=value:%<variable_value> type:%<variable_type> max:%<variable_max> Min:%<variable_min>
  wires:
  ecocoder_calibration9/1 -> Data Type Conversion9/1
  03 process bms output signals/1(sigOutBms_flgConnHv) -> Data Type Conversion10/1
  ecocoder_calibration11/1 -> Data Type Conversion11/1
  Data Type Conversion11/1 -> "Send CAN Message "/3
  Data Type Conversion9/1 -> "Send CAN Message "/1
  Data Type Conversion10/1 -> "Send CAN Message "/2
  Task_Call/1 -> 03 process bms output signals/Trigger
  pwrtrnBmscPack_flgConnReq/1 -> 03 process bms output signals/1(pwrtrnBmscPack_flgConnReq)

== system VHF_central_unit/ASW_Outputs/Command DCDC Converter/Subsystem1 ==
  In1 : Inport
  function : TriggerPort  TriggerType=function-call  VariantControl=(inherit)
  Terminator : Terminator
  wires:
  In1/1 -> Terminator/1

== system VHF_central_unit/ASW_Outputs/Command GenSys/Subsystem1 ==
  In1 : Inport
  function : TriggerPort  TriggerType=function-call  VariantControl=(inherit)
  Terminator : Terminator
  wires:
  In1/1 -> Terminator/1

== system VHF_central_unit/ASW_Outputs/Command Inverter 1/Subsystem1 ==
  In1 : Inport
  function : TriggerPort  TriggerType=function-call  VariantControl=(inherit)
  Terminator : Terminator
  wires:
  In1/1 -> Terminator/1

== system VHF_central_unit/ASW_Outputs/Command Inverter 2/Subsystem1 ==
  In1 : Inport
  function : TriggerPort  TriggerType=function-call  VariantControl=(inherit)
  Terminator : Terminator
  wires:
  In1/1 -> Terminator/1

== system VHF_central_unit/ASW_Powertrain/Command DCDC Converter/Subsystem1 ==
  In1 : Inport
  function : TriggerPort  TriggerType=function-call  VariantControl=(inherit)
  Terminator : Terminator
  wires:
  In1/1 -> Terminator/1

== system VHF_central_unit/ASW_Powertrain/Command GenSys/Subsystem1 ==
  In1 : Inport
  function : TriggerPort  TriggerType=function-call  VariantControl=(inherit)
  Terminator : Terminator
  wires:
  In1/1 -> Terminator/1

== system VHF_central_unit/ASW_Powertrain/Command Inverter 1/Subsystem1 ==
  In1 : Inport
  function : TriggerPort  TriggerType=function-call  VariantControl=(inherit)
  Terminator : Terminator
  wires:
  In1/1 -> Terminator/1

== system VHF_central_unit/ASW_Powertrain/Command Inverter 2/Subsystem1 ==
  In1 : Inport
  function : TriggerPort  TriggerType=function-call  VariantControl=(inherit)
  Terminator : Terminator
  wires:
  In1/1 -> Terminator/1
